simulink library "pm_bulk"  (R2021a)
settings: Solver=VariableStepAuto  StartTime=0.0  StopTime=10.0  RelTol=1e-3
settings Model: Creator=errorput  LastModifiedBy=errorput

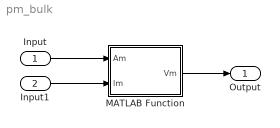
== system pm_bulk ==
  Input : Inport
  Input1 : Inport  Port=2
  MATLAB Function : MATLAB Function  TreatAsAtomicUnit=on
  Output : Outport
  wires:
  Input/1 -> MATLAB Function/1(Am)
  Input1/1 -> MATLAB Function/2(lm)
  MATLAB Function/1(Vm) -> Output/1

== matlab function pm_bulk/MATLAB Function ==
  data: Am input; Vm output; lm input
function Vm  = pm_bulk(Am,lm)
%UNTITLED 计算永磁电机永磁体体积
%   Am    永磁体横截面积
%   lm    永磁体长度
%   Vm    永磁体体积
Vm = Am * lm;
end
